simulink library "battery_monitor_lib"  (R2022b)
settings: Solver=VariableStepAuto  StartTime=0.0  StopTime=10.0  RelTol=1e-3
settings Model: Creator=dr_pa  LastModifiedBy=dr_pa

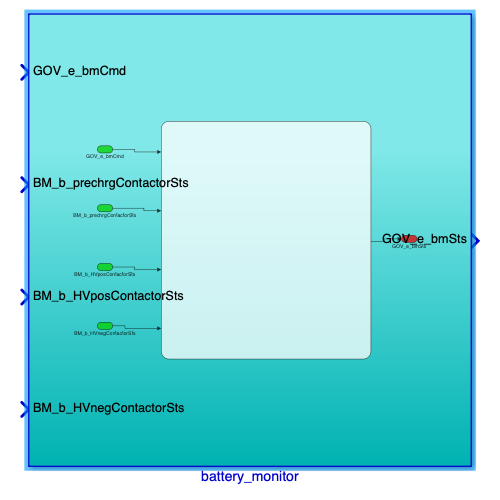
[thumbnail: Simulink's stored preview of the top-level diagram]
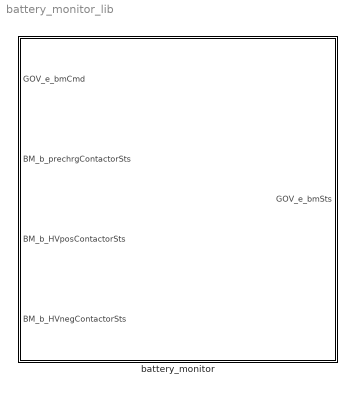
== system battery_monitor_lib ==
  battery_monitor : Subsystem

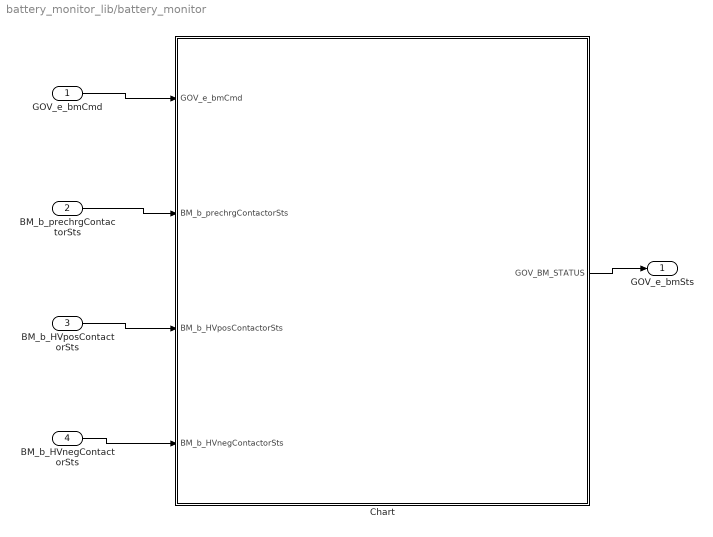
== system battery_monitor_lib/battery_monitor ==
  GOV_e_bmCmd : Inport
  BM_b_prechrgContactorSts : Inport  Port=2
  BM_b_HVposContactorSts : Inport  Port=3
  BM_b_HVnegContactorSts : Inport  Port=4
  Chart : Stateflow chart  TreatAsAtomicUnit=on
  GOV_e_bmSts : Outport
  wires:
  GOV_e_bmCmd/1 -> Chart/1(GOV_e_bmCmd)
  BM_b_prechrgContactorSts/1 -> Chart/2(BM_b_prechrgContactorSts)
  BM_b_HVposContactorSts/1 -> Chart/3(BM_b_HVposContactorSts)
  BM_b_HVnegContactorSts/1 -> Chart/4(BM_b_HVnegContactorSts)
  Chart/1(GOV_BM_STATUS) -> GOV_e_bmSts/1

== stateflow chart battery_monitor_lib/battery_monitor/Chart ==
  state InitialState
    entry:
    GOV_BM_STATUS = BM_INIT;
  state ErrorPrechargeClosedState
    entry:
    GOV_BM_STATUS = ERR_PRECHARGE_CLOSED;
  state ErrorAllClosedState
    entry:
    GOV_BM_STATUS = ERR_ALL_CLOSED;
  state ErrorHVPositive
    entry:
    GOV_BM_STATUS = ERR_HV_POSITIVE;
  state StartupState1
    entry:
    GOV_BM_STATUS = BM_IDLE;
  state StartupState
    entry:
    GOV_BM_STATUS = BM_STARTUP;
  state ErrorStartupState
    entry:
    GOV_BM_STATUS = ERR_STARTUP;
  state InitializePrechargeState
    entry:
    GOV_BM_STATUS = INIT_PRECHARGE;
  state ErrorInitializePrechargeState
    entry:
    GOV_BM_STATUS = ERR_INIT_PRECHARGE;
  state PrechargeState
    entry:
    GOV_BM_STATUS = PRECHARGE;
  state ErrorPrechargeState
    entry:
    GOV_BM_STATUS = ERR_PRECHARGE;
  state RunningState
    entry:
    GOV_BM_STATUS = BM_RUNNING;
  state ErrorRunningState
    entry:
    GOV_BM_STATUS = ERR_RUNNING;
  (default) -> InitialState
  InitialState -> PrechargeState [order 5] : [BM_b_prechrgContactorSts == 1 && BM_b_HVnegContactorSts == 1 && BM_b_HVposContactorSts == 0]
  InitialState -> RunningState [order 6] : [BM_b_prechrgContactorSts == 0 && BM_b_HVnegContactorSts == 1 && BM_b_HVposContactorSts == 1]
  InitialState -> ErrorPrechargeClosedState [order 2] : [BM_b_prechrgContactorSts == 1 && BM_b_HVnegContactorSts == 0 && BM_b_HVposContactorSts == 0]
  InitialState -> StartupState1 [order 1] : [BM_b_prechrgContactorSts == 0 && BM_b_HVnegContactorSts == 0 && BM_b_HVposContactorSts == 0]
  InitialState -> ErrorAllClosedState [order 3] : [BM_b_prechrgContactorSts == 1 && BM_b_HVnegContactorSts == 1 && BM_b_HVposContactorSts == 1]
  InitialState -> ErrorHVPositive [order 4] : [BM_b_prechrgContactorSts == 0 && BM_b_HVnegContactorSts == 0 && BM_b_HVposContactorSts == 1]
  StartupState1 -> StartupState : [BM_b_prechrgContactorSts == 0 && BM_b_HVnegContactorSts == 1 && BM_b_HVposContactorSts == 0]
  StartupState -> ErrorStartupState [order 2] : after(1,sec)
  StartupState -> InitializePrechargeState [order 1] : [BM_b_prechrgContactorSts == 1 && BM_b_HVnegContactorSts == 1 && BM_b_HVposContactorSts == 0]
  InitializePrechargeState -> ErrorInitializePrechargeState [order 2] : after(1,sec)
  InitializePrechargeState -> PrechargeState [order 1] : [BM_b_prechrgContactorSts == 1 && BM_b_HVnegContactorSts == 1 && BM_b_HVposContactorSts == 1]
  PrechargeState -> ErrorPrechargeState [order 2] : after(1,sec)
  PrechargeState -> RunningState [order 1] : [BM_b_prechrgContactorSts == 0 && BM_b_HVnegContactorSts == 1 && BM_b_HVposContactorSts == 1]
  RunningState -> ErrorRunningState [order 2] : after(1,sec)
  RunningState -> RunningState [order 1] : [BM_b_prechrgContactorSts == 0 && BM_b_HVnegContactorSts == 1 && BM_b_HVposContactorSts == 1]
  data: GOV_e_bmCmd input; BM_b_prechrgContactorSts input; BM_b_HVposContactorSts input; BM_b_HVnegContactorSts input; GOV_BM_STATUS output Enum: BM_STATUSES
